simulink model "f16_6dof3"  (R2020b)
settings: Solver=VariableStepAuto  StartTime=0.0  StopTime=100  RelTol=1e-3
values from neighbouring files (symbols this model uses):
  b = 9.144    [f16_script3.m]
  chord = 3.45    [f16_script3.m]
  d_r = 0    [f16_script3.m]
  d_SB = 0    [f16_script3.m]
  h_ref = 0    [f16_script3.m]
  Mass = 9300    [f16_script3.m]
  phi_c = 10    [f16_script3.m]
  S = 27.88    [f16_script3.m]
  V_c = 153    [f16_script3.m]
  X_cg = 0.35    [f16_script3.m]
  X_cg_ref = 0.35    [f16_script3.m]
undefined symbols (not defined in the file or in its folder): block, Earth, f16, f16_database, WGS84
libraries: simulink_extras x7, slpidlib x4, aerolibfltsims x2, shared6dof x1, aerolibatmos2 x1, aerolibasang x1, aerolibtransform2 x1
(part 1 of 2)
settings Model: Creator=celal  LastModifiedBy=celal

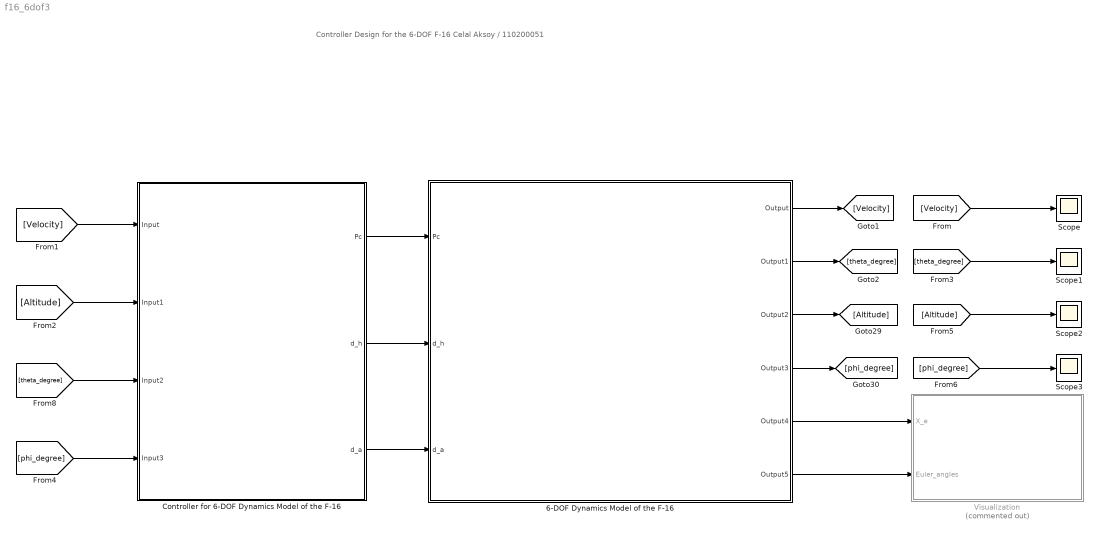
== system f16_6dof3 ==
  note: Controller Design for the 6-DOF F-16
      |
      | Celal Aksoy / 110200051
  " 6-DOF Dynamics Model of the F-16" : Subsystem
  Controller for 6-DOF Dynamics Model of the F-16 : Subsystem
  Scope{,1..3} (4 alike) : Scope
  Visualization : Subsystem  Commented=on
  wires:
  " 6-DOF Dynamics Model of the F-16"/1(Output) -> [Velocity]
  " 6-DOF Dynamics Model of the F-16"/2(Output1) -> [theta_degree]
  " 6-DOF Dynamics Model of the F-16"/3(Output2) -> [Altitude]
  " 6-DOF Dynamics Model of the F-16"/4(Output3) -> [phi_degree]
  [Velocity] -> Controller for 6-DOF Dynamics Model of the F-16/1(Input)
  [theta_degree] -> Controller for 6-DOF Dynamics Model of the F-16/3(Input2)
  [phi_degree] -> Controller for 6-DOF Dynamics Model of the F-16/4(Input3)
  [Altitude] -> Controller for 6-DOF Dynamics Model of the F-16/2(Input1)
  [Velocity] -> Scope/1
  [Altitude] -> Scope2/1
  [phi_degree] -> Scope3/1
  [theta_degree] -> Scope1/1
  Controller for 6-DOF Dynamics Model of the F-16/2(d_h) -> " 6-DOF Dynamics Model of the F-16"/2(d_h)
  Controller for 6-DOF Dynamics Model of the F-16/1(Pc) -> " 6-DOF Dynamics Model of the F-16"/1(Pc)
  Controller for 6-DOF Dynamics Model of the F-16/3(d_a) -> " 6-DOF Dynamics Model of the F-16"/3(d_a)
  " 6-DOF Dynamics Model of the F-16"/5(Output4) -> Visualization/1(X_e)
  " 6-DOF Dynamics Model of the F-16"/6(Output5) -> Visualization/2(Euler_angles)

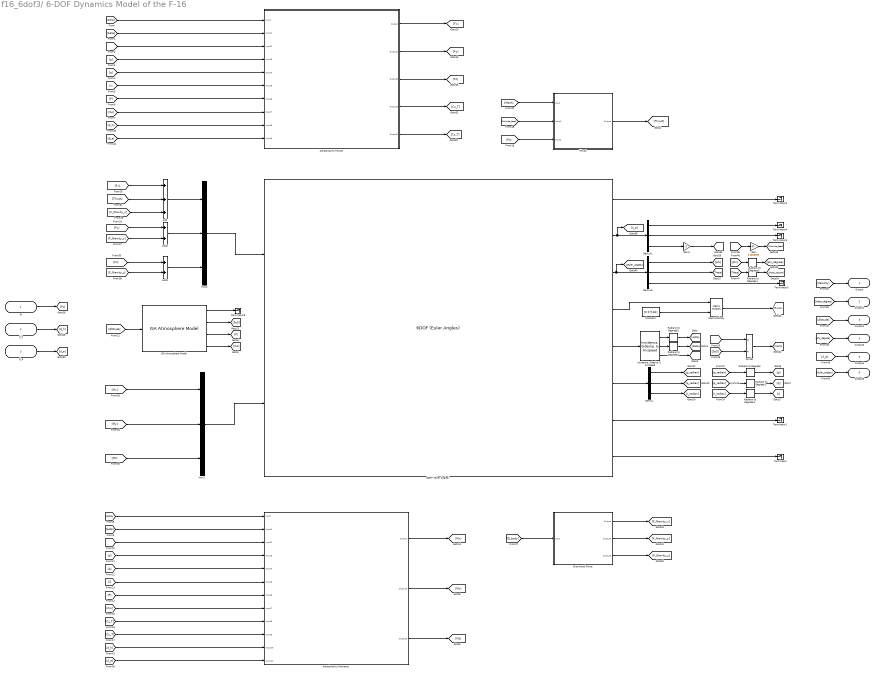
== system f16_6dof3/ 6-DOF Dynamics Model of the F-16 ==
  Pc : Inport
  d_h : Inport  Port=2
  d_a : Inport  Port=3
  6DOF (Euler Angles) : shared6dof/6DOF (Euler Angles)  units=Metric (MKS)  mtype=Fixed  rep=Euler Angles  xme_0=[0, 0, -3048 ]  Vm_0=[131.2, 0, 0]  eul_0=[0, 0, 0]  pm_0=[0, 0, 0]  mass_0=9300  mass_e=0.5  mass_f=2.0  inertia=I  inertia_e=eye(3)  inertia_f=2*eye(3)  k_quat=1.0  vre_flag=on  abi_flag=off  aMode=0  xme_statename=''  Vm_statename=''  eul_statename=''  quat_statename=''  pm_statename=''  mass_statename=''
      settings: SourceProductBaseCode=AE,PW,MT,UV,VE,VP
  Add : Sum  Inputs=+++
  Add1 : Sum
  Add3 : Sum
  Aerodynamic Forces : Subsystem
  Aerodynamic Moments : Subsystem
  Constant : Constant  Value=[0 0 9.81]
  Demux : Demux  Outputs=3
  Demux1 : Demux  Outputs=3
  Demux3 : Demux  Outputs=3
  Divide : Product  Inputs=*/
  Gain : Gain  Gain=3.2808399
  Gain1 : Gain  Gain=-1
  Gravitional Force : Subsystem
  ISA Atmosphere Model : aerolibatmos2/ISA Atmosphere Model  custom=off  g=9.80665  gamma=1.4  R=287.0531  L=0.0065  h_trop=11000  h_strat=20000  rho0=1.225  P0=101325  T0=288.15  h0=0
  "Incidence, Sideslip, & Airspeed" : aerolibasang/Incidence, Sideslip, & Airspeed
  MatrixMultiply : Product  Multiplication=Matrix(*)
  Mux1 : Mux  Inputs=3
  Mux2 : Mux  Inputs=3
  Radians to Degrees{,1..6} (7 alike) : simulink_extras/Transformations/Radians to Degrees
  Terminator{,1..5,8} (7 alike) : Terminator
  Thrust : Subsystem
  Output : Outport
  Output1 : Outport  Port=2
  Output2 : Outport  Port=3
  Output3 : Outport  Port=4
  Output4 : Outport  Port=5
  Output5 : Outport  Port=6
  wires:
  Gain/1 -> [Altitude_feet]
  [P] -> Aerodynamic Forces/7(Input6)
  6DOF (Euler Angles)/5 -> "Incidence, Sideslip, & Airspeed"/1
  [beta] -> Aerodynamic Forces/2(Input1)
  [beta] -> Aerodynamic Moments/2(Input1)
  Aerodynamic Moments/1(Output) -> [Mx]
  ISA Atmosphere Model/4 -> [rho]
  [Mz] -> Mux1/3
  [alpha] -> Aerodynamic Forces/1(Input)
  Demux/1 -> [p_radian]
  [r] -> Aerodynamic Forces/6(Input5)
  Demux3/2 -> [Theta]
  Mux1/1 -> 6DOF (Euler Angles)/2
  Demux/3 -> [r_radian]
  Demux/2 -> [q_radian]
  [r] -> Aerodynamic Moments/6(Input5)
  Constant/1 -> MatrixMultiply/2
  6DOF (Euler Angles)/7 -> Terminator1/1
  [rho] -> Aerodynamic Forces/8(Input7)
  [Altitude_feet] -> Thrust/2(Input1)
  ISA Atmosphere Model/3 -> [P]
  6DOF (Euler Angles)/6 -> Demux/1
  [r_radian] -> Radians to Degrees2/1
  [p] -> Aerodynamic Forces/4(Input3)
  ISA Atmosphere Model/2 -> [SoS]
  [G_body] -> Gravitional Force/1(Input)
  [Mach] -> Thrust/1(Input)
  Demux1/1 -> Terminator4/1
  [rho] -> Aerodynamic Moments/8(Input7)
  Aerodynamic Forces/1(Output) -> [Fx]
  [P] -> Aerodynamic Moments/7(Input6)
  [Cz_T] -> Aerodynamic Moments/9(Input8)
  Aerodynamic Moments/3(Output2) -> [Mz]
  [p_radian] -> Radians to Degrees/1
  Thrust/1(Output) -> [Thrust]
  [alpha] -> Aerodynamic Moments/1(Input)
  Aerodynamic Moments/2(Output1) -> [My]
  [Velocity] -> Aerodynamic Moments/3(Input2)
  Aerodynamic Forces/3(Output2) -> [Fz]
  [q] -> Aerodynamic Forces/5(Input4)
  Radians to Degrees2/1 -> [r]
  [q_radian] -> Radians to Degrees1/1
  Radians to Degrees1/1 -> [q]
  [p] -> Aerodynamic Moments/4(Input3)
  6DOF (Euler Angles)/2 -> [X_e], Demux1/1
  MatrixMultiply/1 -> [G_body]
  Divide/1 -> [Mach]
  6DOF (Euler Angles)/3 -> [Euler_angles], Demux3/1
  6DOF (Euler Angles)/1 -> Terminator2/1
  6DOF (Euler Angles)/8 -> Terminator/1
  Demux1/2 -> Terminator5/1
  [Altitude] -> ISA Atmosphere Model/1
  [SoS] -> Divide/2
  [Cy_T] -> Aerodynamic Moments/10(Input9)
  [q] -> Aerodynamic Moments/5(Input4)
  Aerodynamic Forces/2(Output1) -> [Fy]
  [Mx] -> Mux1/1
  ISA Atmosphere Model/1 -> Terminator8/1
  [Velocity] -> Aerodynamic Forces/3(Input2)
  [My] -> Mux1/2
  [Altitude] -> Gain/1
  Radians to Degrees/1 -> [p]
  6DOF (Euler Angles)/4 -> MatrixMultiply/1
  [Velocity] -> Divide/1
  Demux3/3 -> Terminator3/1
  Demux3/1 -> [phi]
  [Pc] -> Thrust/3(Input2)
  Gravitional Force/2(Output1) -> [F_Gravity_y]
  Gravitional Force/3(Output2) -> [F_Gravity_z]
  Gravitional Force/1(Output) -> [F_Gravity_x]
  Pc/1 -> [Pc]
  [Velocity] -> Output/1
  d_h/1 -> [d_h]
  [d_h] -> Aerodynamic Forces/9(Input8)
  [d_h] -> Aerodynamic Moments/11(Input10)
  [Altitude] -> Output2/1
  [phi_degree] -> Output3/1
  d_a/1 -> [d_a]
  [d_a] -> Aerodynamic Forces/10(Input9)
  [d_a] -> Aerodynamic Moments/12(Input11)
  Aerodynamic Forces/4(Output3) -> [Cz_T]
  Aerodynamic Forces/5(Output4) -> [Cy_T]
  [phi] -> Radians to Degrees3/1
  [Theta] -> Radians to Degrees4/1
  Radians to Degrees3/1 -> [phi_degree]
  Radians to Degrees4/1 -> [theta_degree]
  [theta_degree] -> Output1/1
  Gain1/1 -> [Altitude]
  Mux2/1 -> 6DOF (Euler Angles)/1
  [Fx] -> Add/1
  [Thrust] -> Add/2
  [F_Gravity_x] -> Add/3
  Add/1 -> Mux2/1
  [Fy] -> Add1/1
  [F_Gravity_y] -> Add1/2
  Add1/1 -> Mux2/2
  Add3/1 -> Mux2/3
  [Fz] -> Add3/1
  [F_Gravity_z] -> Add3/2
  Demux1/3 -> Gain1/1
  "Incidence, Sideslip, & Airspeed"/1 -> Radians to Degrees5/1
  "Incidence, Sideslip, & Airspeed"/2 -> Radians to Degrees6/1
  Radians to Degrees5/1 -> [alpha]
  Radians to Degrees6/1 -> [beta]
  "Incidence, Sideslip, & Airspeed"/3 -> [Velocity]
  [X_e] -> Output4/1
  [Euler_angles] -> Output5/1

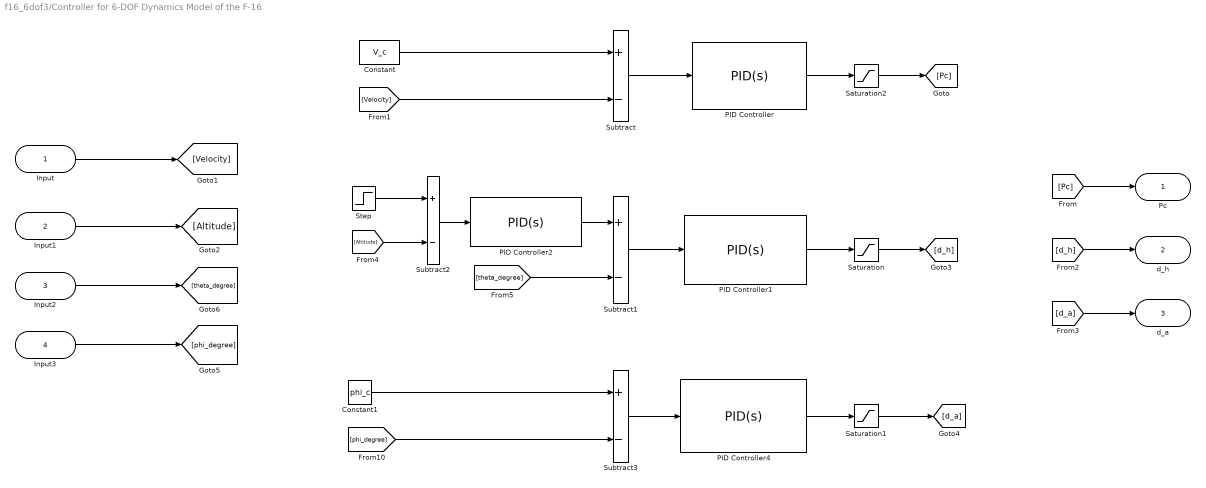
== system f16_6dof3/Controller for 6-DOF Dynamics Model of the F-16 ==
  Input : Inport
  Input1 : Inport  Port=2
  Input2 : Inport  Port=3
  Input3 : Inport  Port=4
  Constant : Constant  Value=V_c
  Constant1 : Constant  Value=phi_c
  PID Controller : slpidlib/PID Controller  Controller=PID  Form=Parallel  TimeDomain=Continuous-time  UseExternalTs=off  SampleTime=-1  IntegratorMethod=Forward Euler  FilterMethod=Forward Euler  ControllerParametersSource=internal  P=70  I=15  D=50  UseFilter=on  N=10  TunerSelectOption=Transfer Function Based (PID Tuner App)  InitialConditionSource=internal  InitialConditionForIntegrator=0  InitialConditionForFilter=0  DifferentiatorICPrevScaledInput=0  ExternalReset=none  TrackingMode=off  Kt=1  LimitOutput=off  SatLimitsSource=internal  UpperSaturationLimit=inf  LowerSaturationLimit=-inf  LinearizeAsGain=on  AntiWindupMode=none  Kb=1  POutMin=[]  POutMax=[]  IOutMin=[]  IOutMax=[]  DOutMin=[]  DOutMax=[]  NOutMin=[]  NOutMax=[]  SumOutMin=[]  SumOutMax=[]  SaturationOutMin=[]  SaturationOutMax=[]  PParamMin=[]  PParamMax=[]  IParamMin=[]  IParamMax=[]  DParamMin=[]  DParamMax=[]  NParamMin=[]  NParamMax=[]  KbParamMin=[]  KbParamMax=[]  KtParamMin=[]  KtParamMax=[]  KbOutMin=[]  KbOutMax=[]  KtOutMin=[]  KtOutMax=[]  IntegratorOutMin=[]  IntegratorOutMax=[]  FilterOutMin=[]  FilterOutMax=[]  SumI1OutMin=[]  SumI1OutMax=[]  SumI2OutMin=[]  SumI2OutMax=[]  SumI3OutMin=[]  SumI3OutMax=[]  SumI4OutMin=[]  SumI4OutMax=[]  SumDOutMin=[]  SumDOutMax=[]  DifferentiatorOutMin=[]  DifferentiatorOutMax=[]  FilterDiffOutCoefMin=[]  FilterDiffOutCoefMax=[]  ReciprocalOutMin=[]  ReciprocalOutMax=[]  SumDenOutMin=[]  SumDenOutMax=[]  SumNumOutMin=[]  SumNumOutMax=[]  DivideOutMin=[]  DivideOutMax=[]  UdiffTsProdOutMin=[]  UdiffTsProdOutMax=[]  NTsProdOutMin=[]  NTsProdOutMax=[]  UintegralTsProdOutMin=[]  UintegralTsProdOutMax=[]  UngainTsProdOutMin=[]  UngainTsProdOutMax=[]  IntegratorContinuousStateAttributes=''  IntegratorStateMustResolveToSignalObject=off  IntegratorRTWStateStorageClass=Auto  FilterContinuousStateAttributes=''  FilterStateMustResolveToSignalObject=off  FilterRTWStateStorageClass=Auto  ParallelPVariant=InternalParameters  IdealPVariant=Disabled  IVariant=InternalParameters  DVariant=InternalParameters  IntegratorVariant=Continuous  SatVariant=Disabled  AWVariant=Passthrough  PCopyVariant=Disabled  TRVariant=Disabled  FdbkBlocksVariant=Forward  IdealPFdbkVariant=Disabled  SatFdbkVariant=Disabled  DerivativeFilterVariant=ContFilter  NVariant=InternalParameters  NCopyVariant=Disabled  FilterICVariant=InternalICsFilter  IntegratorICVariant=InternalICs  ExternalResetVariant=Disabled  TRSumVariant=Passthrough  SumFdbkVariant=Disabled  SumVariant=Sum_PID  TsampFilterVariant=InternalTs  TsampNgainVariant=Passthrough  TsampIntegralVariant=Passthrough  ExternalSaturationOutDataTypeStr=Inherit: Same as second input  mask(PID 1dof){}
      mask Display:
      | % This is a new mask on top of the base mask.
      | % Use "View base mask" link below to see the base mask.
      | disp("Velocity Hold Controller");
  PID Controller1 : slpidlib/PID Controller  Controller=PID  Form=Parallel  TimeDomain=Continuous-time  UseExternalTs=off  SampleTime=-1  IntegratorMethod=Forward Euler  FilterMethod=Forward Euler  ControllerParametersSource=internal  P=-6e-07  I=-3e-10  D=-12e-7  UseFilter=on  N=2.9  TunerSelectOption=Transfer Function Based (PID Tuner App)  InitialConditionSource=internal  InitialConditionForIntegrator=0  InitialConditionForFilter=0  DifferentiatorICPrevScaledInput=0  ExternalReset=none  TrackingMode=off  Kt=1  LimitOutput=off  SatLimitsSource=internal  UpperSaturationLimit=inf  LowerSaturationLimit=-inf  LinearizeAsGain=on  AntiWindupMode=none  Kb=1  POutMin=[]  POutMax=[]  IOutMin=[]  IOutMax=[]  DOutMin=[]  DOutMax=[]  NOutMin=[]  NOutMax=[]  SumOutMin=[]  SumOutMax=[]  SaturationOutMin=[]  SaturationOutMax=[]  PParamMin=[]  PParamMax=[]  IParamMin=[]  IParamMax=[]  DParamMin=[]  DParamMax=[]  NParamMin=[]  NParamMax=[]  KbParamMin=[]  KbParamMax=[]  KtParamMin=[]  KtParamMax=[]  KbOutMin=[]  KbOutMax=[]  KtOutMin=[]  KtOutMax=[]  IntegratorOutMin=[]  IntegratorOutMax=[]  FilterOutMin=[]  FilterOutMax=[]  SumI1OutMin=[]  SumI1OutMax=[]  SumI2OutMin=[]  SumI2OutMax=[]  SumI3OutMin=[]  SumI3OutMax=[]  SumI4OutMin=[]  SumI4OutMax=[]  SumDOutMin=[]  SumDOutMax=[]  DifferentiatorOutMin=[]  DifferentiatorOutMax=[]  FilterDiffOutCoefMin=[]  FilterDiffOutCoefMax=[]  ReciprocalOutMin=[]  ReciprocalOutMax=[]  SumDenOutMin=[]  SumDenOutMax=[]  SumNumOutMin=[]  SumNumOutMax=[]  DivideOutMin=[]  DivideOutMax=[]  UdiffTsProdOutMin=[]  UdiffTsProdOutMax=[]  NTsProdOutMin=[]  NTsProdOutMax=[]  UintegralTsProdOutMin=[]  UintegralTsProdOutMax=[]  UngainTsProdOutMin=[]  UngainTsProdOutMax=[]  IntegratorContinuousStateAttributes=''  IntegratorStateMustResolveToSignalObject=off  IntegratorRTWStateStorageClass=Auto  FilterContinuousStateAttributes=''  FilterStateMustResolveToSignalObject=off  FilterRTWStateStorageClass=Auto  ParallelPVariant=InternalParameters  IdealPVariant=Disabled  IVariant=InternalParameters  DVariant=InternalParameters  IntegratorVariant=Continuous  SatVariant=Disabled  AWVariant=Passthrough  PCopyVariant=Disabled  TRVariant=Disabled  FdbkBlocksVariant=Forward  IdealPFdbkVariant=Disabled  SatFdbkVariant=Disabled  DerivativeFilterVariant=ContFilter  NVariant=InternalParameters  NCopyVariant=Disabled  FilterICVariant=InternalICsFilter  IntegratorICVariant=InternalICs  ExternalResetVariant=Disabled  TRSumVariant=Passthrough  SumFdbkVariant=Disabled  SumVariant=Sum_PID  TsampFilterVariant=InternalTs  TsampNgainVariant=Passthrough  TsampIntegralVariant=Passthrough  ExternalSaturationOutDataTypeStr=Inherit: Same as second input  mask(PID 1dof){}
      mask Display:
      | % This is a new mask on top of the base mask.
      | % Use "View base mask" link below to see the base mask.
      | disp("Pitch-Attitude Hold Controller")
  PID Controller2 : slpidlib/PID Controller  Controller=PID  Form=Parallel  TimeDomain=Continuous-time  UseExternalTs=off  SampleTime=-1  IntegratorMethod=Forward Euler  FilterMethod=Forward Euler  ControllerParametersSource=internal  P=10000000  I=50000  D=1000  UseFilter=on  N=1e-03  TunerSelectOption=Transfer Function Based (PID Tuner App)  InitialConditionSource=internal  InitialConditionForIntegrator=0  InitialConditionForFilter=0  DifferentiatorICPrevScaledInput=0  ExternalReset=none  TrackingMode=off  Kt=1  LimitOutput=off  SatLimitsSource=internal  UpperSaturationLimit=inf  LowerSaturationLimit=-inf  LinearizeAsGain=on  AntiWindupMode=none  Kb=1  POutMin=[]  POutMax=[]  IOutMin=[]  IOutMax=[]  DOutMin=[]  DOutMax=[]  NOutMin=[]  NOutMax=[]  SumOutMin=[]  SumOutMax=[]  SaturationOutMin=[]  SaturationOutMax=[]  PParamMin=[]  PParamMax=[]  IParamMin=[]  IParamMax=[]  DParamMin=[]  DParamMax=[]  NParamMin=[]  NParamMax=[]  KbParamMin=[]  KbParamMax=[]  KtParamMin=[]  KtParamMax=[]  KbOutMin=[]  KbOutMax=[]  KtOutMin=[]  KtOutMax=[]  IntegratorOutMin=[]  IntegratorOutMax=[]  FilterOutMin=[]  FilterOutMax=[]  SumI1OutMin=[]  SumI1OutMax=[]  SumI2OutMin=[]  SumI2OutMax=[]  SumI3OutMin=[]  SumI3OutMax=[]  SumI4OutMin=[]  SumI4OutMax=[]  SumDOutMin=[]  SumDOutMax=[]  DifferentiatorOutMin=[]  DifferentiatorOutMax=[]  FilterDiffOutCoefMin=[]  FilterDiffOutCoefMax=[]  ReciprocalOutMin=[]  ReciprocalOutMax=[]  SumDenOutMin=[]  SumDenOutMax=[]  SumNumOutMin=[]  SumNumOutMax=[]  DivideOutMin=[]  DivideOutMax=[]  UdiffTsProdOutMin=[]  UdiffTsProdOutMax=[]  NTsProdOutMin=[]  NTsProdOutMax=[]  UintegralTsProdOutMin=[]  UintegralTsProdOutMax=[]  UngainTsProdOutMin=[]  UngainTsProdOutMax=[]  IntegratorContinuousStateAttributes=''  IntegratorStateMustResolveToSignalObject=off  IntegratorRTWStateStorageClass=Auto  FilterContinuousStateAttributes=''  FilterStateMustResolveToSignalObject=off  FilterRTWStateStorageClass=Auto  ParallelPVariant=InternalParameters  IdealPVariant=Disabled  IVariant=InternalParameters  DVariant=InternalParameters  IntegratorVariant=Continuous  SatVariant=Disabled  AWVariant=Passthrough  PCopyVariant=Disabled  TRVariant=Disabled  FdbkBlocksVariant=Forward  IdealPFdbkVariant=Disabled  SatFdbkVariant=Disabled  DerivativeFilterVariant=ContFilter  NVariant=InternalParameters  NCopyVariant=Disabled  FilterICVariant=InternalICsFilter  IntegratorICVariant=InternalICs  ExternalResetVariant=Disabled  TRSumVariant=Passthrough  SumFdbkVariant=Disabled  SumVariant=Sum_PID  TsampFilterVariant=InternalTs  TsampNgainVariant=Passthrough  TsampIntegralVariant=Passthrough  ExternalSaturationOutDataTypeStr=Inherit: Same as second input  mask(PID 1dof){}
      mask Display:
      | % This is a new mask on top of the base mask.
      | % Use "View base mask" link below to see the base mask.
      | disp("Altitude Hold Controller");
  PID Controller4 : slpidlib/PID Controller  Controller=PID  Form=Parallel  TimeDomain=Continuous-time  UseExternalTs=off  SampleTime=-1  IntegratorMethod=Forward Euler  FilterMethod=Forward Euler  ControllerParametersSource=internal  P=-15  I=-0.010  D=-0.001  UseFilter=on  N=0.6  TunerSelectOption=Transfer Function Based (PID Tuner App)  InitialConditionSource=internal  InitialConditionForIntegrator=0  InitialConditionForFilter=0  DifferentiatorICPrevScaledInput=0  ExternalReset=none  TrackingMode=off  Kt=1  LimitOutput=off  SatLimitsSource=internal  UpperSaturationLimit=inf  LowerSaturationLimit=-inf  LinearizeAsGain=on  AntiWindupMode=none  Kb=1  POutMin=[]  POutMax=[]  IOutMin=[]  IOutMax=[]  DOutMin=[]  DOutMax=[]  NOutMin=[]  NOutMax=[]  SumOutMin=[]  SumOutMax=[]  SaturationOutMin=[]  SaturationOutMax=[]  PParamMin=[]  PParamMax=[]  IParamMin=[]  IParamMax=[]  DParamMin=[]  DParamMax=[]  NParamMin=[]  NParamMax=[]  KbParamMin=[]  KbParamMax=[]  KtParamMin=[]  KtParamMax=[]  KbOutMin=[]  KbOutMax=[]  KtOutMin=[]  KtOutMax=[]  IntegratorOutMin=[]  IntegratorOutMax=[]  FilterOutMin=[]  FilterOutMax=[]  SumI1OutMin=[]  SumI1OutMax=[]  SumI2OutMin=[]  SumI2OutMax=[]  SumI3OutMin=[]  SumI3OutMax=[]  SumI4OutMin=[]  SumI4OutMax=[]  SumDOutMin=[]  SumDOutMax=[]  DifferentiatorOutMin=[]  DifferentiatorOutMax=[]  FilterDiffOutCoefMin=[]  FilterDiffOutCoefMax=[]  ReciprocalOutMin=[]  ReciprocalOutMax=[]  SumDenOutMin=[]  SumDenOutMax=[]  SumNumOutMin=[]  SumNumOutMax=[]  DivideOutMin=[]  DivideOutMax=[]  UdiffTsProdOutMin=[]  UdiffTsProdOutMax=[]  NTsProdOutMin=[]  NTsProdOutMax=[]  UintegralTsProdOutMin=[]  UintegralTsProdOutMax=[]  UngainTsProdOutMin=[]  UngainTsProdOutMax=[]  IntegratorContinuousStateAttributes=''  IntegratorStateMustResolveToSignalObject=off  IntegratorRTWStateStorageClass=Auto  FilterContinuousStateAttributes=''  FilterStateMustResolveToSignalObject=off  FilterRTWStateStorageClass=Auto  ParallelPVariant=InternalParameters  IdealPVariant=Disabled  IVariant=InternalParameters  DVariant=InternalParameters  IntegratorVariant=Continuous  SatVariant=Disabled  AWVariant=Passthrough  PCopyVariant=Disabled  TRVariant=Disabled  FdbkBlocksVariant=Forward  IdealPFdbkVariant=Disabled  SatFdbkVariant=Disabled  DerivativeFilterVariant=ContFilter  NVariant=InternalParameters  NCopyVariant=Disabled  FilterICVariant=InternalICsFilter  IntegratorICVariant=InternalICs  ExternalResetVariant=Disabled  TRSumVariant=Passthrough  SumFdbkVariant=Disabled  SumVariant=Sum_PID  TsampFilterVariant=InternalTs  TsampNgainVariant=Passthrough  TsampIntegralVariant=Passthrough  ExternalSaturationOutDataTypeStr=Inherit: Same as second input  mask(PID 1dof){}
      mask Display:
      | % This is a new mask on top of the base mask.
      | % Use "View base mask" link below to see the base mask.
      | disp("Roll-Angle Hold Controller")
  Saturation : Saturate  UpperLimit=25  LowerLimit=-25
  Saturation1 : Saturate  UpperLimit=20  LowerLimit=-20
  Saturation2 : Saturate  UpperLimit=100  LowerLimit=0
  Step : Step  Time=60  Before=10100*0.3048  After=9090*0.3048  SampleTime=0
  Subtract{,1..3} (4 alike) : Sum  Inputs=+-
  Pc : Outport
  d_h : Outport  Port=2
  d_a : Outport  Port=3
  wires:
  Constant/1 -> Subtract/1
  Saturation/1 -> [d_h]
  PID Controller4/1 -> Saturation1/1
  Subtract3/1 -> PID Controller4/1
  Saturation1/1 -> [d_a]
  PID Controller2/1 -> Subtract1/1
  Subtract2/1 -> PID Controller2/1
  PID Controller1/1 -> Saturation/1
  [phi_degree] -> Subtract3/2
  Step/1 -> Subtract2/1
  Subtract/1 -> PID Controller/1
  [Altitude] -> Subtract2/2
  Constant1/1 -> Subtract3/1
  Subtract1/1 -> PID Controller1/1
  [theta_degree] -> Subtract1/2
  [Velocity] -> Subtract/2
  Saturation2/1 -> [Pc]
  PID Controller/1 -> Saturation2/1
  Input3/1 -> [phi_degree]
  Input2/1 -> [theta_degree]
  Input1/1 -> [Altitude]
  Input/1 -> [Velocity]
  [Pc] -> Pc/1
  [d_h] -> d_h/1
  [d_a] -> d_a/1

== system f16_6dof3/Visualization ==
  X_e : Inport
  Euler_angles : Inport  Port=2
  Constant : Constant  Value=h_ref
  Demux : Demux  Outputs=3
  Demux1 : Demux  Outputs=2
  Flat Earth to LLA : aerolibtransform2/Flat Earth to LLA  units=Metric (MKS)  ptype=Earth (WGS84)  F=1/298.257223563  R=6378137  refPosPort=off  LL0=[0 10]  psi=0
  FlightGear Preconfigured 6DoF Animation : aerolibfltsims/FlightGear Preconfigured 6DoF Animation  xFlightGearVersion=v2019.1  DestinationIpAddress=127.0.0.1  DestinationPort=5502  SampleTime=1/30  packetVersion=24
  Generate Run Script : aerolibfltsims/Generate Run Script  Architecture=Default  dataFlow=Send  GeometryModelName=f16-block-30  AirportId=KSFO  RunwayId=10L  InitialAltitude=7224  InitialHeading=113  OffsetDistance=4.72  OffsetAzimuth=0  InstallScenery=off  DisableShaders=off  OriginAddress=127.0.0.1  DestinationPort=5502  OriginPort=5505  LocalAddress=127.0.0.1  OutputFileName=runfg.bat  FlightGearBaseDirectory=C:\Program Files\FlightGear 2020.3
  Mux : Mux  Inputs=6
  wires:
  Constant/1 -> Flat Earth to LLA/2
  Mux/1 -> FlightGear Preconfigured 6DoF Animation/1
  Demux/1 -> Mux/4
  [X_e] -> Flat Earth to LLA/1
  Demux/2 -> Mux/5
  [Euler_angles] -> Demux/1
  Demux/3 -> Mux/6
  X_e/1 -> [X_e]
  Euler_angles/1 -> [Euler_angles]
  Flat Earth to LLA/1 -> Demux1/1
  Demux1/2 -> Mux/1
  Demux1/1 -> Mux/2
  Flat Earth to LLA/2 -> Mux/3

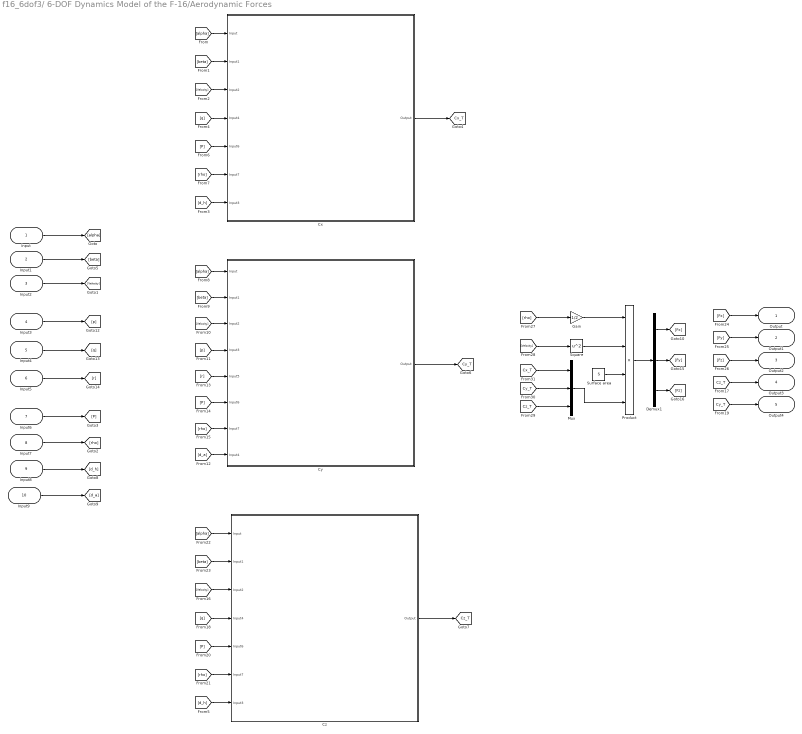
== system f16_6dof3/ 6-DOF Dynamics Model of the F-16/Aerodynamic Forces ==
  Input : Inport
  Input1 : Inport  Port=2
  Input2 : Inport  Port=3
  Input3 : Inport  Port=4
  Input4 : Inport  Port=5
  Input5 : Inport  Port=6
  Input6 : Inport  Port=7
  Input7 : Inport  Port=8
  Input8 : Inport  Port=9
  Input9 : Inport  Port=10
  Cx : Subsystem
  Cy : Subsystem
  Cz : Subsystem
  Demux1 : Demux  Outputs=3
  Gain : Gain  Gain=1/2
  Mux : Mux  Inputs=3
  Product : Product  Inputs=4
  Square : Math  Operator=square  SaturateOnIntegerOverflow=on
  Surface area : Constant  Value=S
  Output : Outport
  Output1 : Outport  Port=2
  Output2 : Outport  Port=3
  Output3 : Outport  Port=4
  Output4 : Outport  Port=5
  tag scope: Cx_T=global, Cy_T=global, Cz_T=global
  wires:
  Input/1 -> [alpha]
  Input1/1 -> [beta]
  Input2/1 -> [Velocity]
  Input6/1 -> [P]
  Input7/1 -> [rho]
  Input5/1 -> [r]
  Input4/1 -> [q]
  Input3/1 -> [p]
  [alpha] -> Cx/1(Input)
  [beta] -> Cx/2(Input1)
  [Velocity] -> Cx/3(Input2)
  [q] -> Cx/4(Input4)
  [P] -> Cx/5(Input6)
  [rho] -> Cx/6(Input7)
  Cx/1(Output) -> [Cx_T]
  Cy/1(Output) -> [Cy_T]
  [P] -> Cy/6(Input6)
  [Velocity] -> Cy/3(Input2)
  [rho] -> Cy/7(Input7)
  [alpha] -> Cy/1(Input)
  [beta] -> Cy/2(Input1)
  [p] -> Cy/4(Input3)
  [r] -> Cy/5(Input5)
  [q] -> Cz/4(Input4)
  [beta] -> Cz/2(Input1)
  [alpha] -> Cz/1(Input)
  [rho] -> Cz/6(Input7)
  [Velocity] -> Cz/3(Input2)
  [P] -> Cz/5(Input6)
  Cz/1(Output) -> [Cz_T]
  [Fx] -> Output/1
  [Fy] -> Output1/1
  [Fz] -> Output2/1
  Demux1/3 -> [Fz]
  Surface area/1 -> Product/3
  Demux1/1 -> [Fx]
  Square/1 -> Product/2
  Gain/1 -> Product/1
  [Velocity] -> Square/1
  [Cx_T] -> Mux/1
  [rho] -> Gain/1
  Demux1/2 -> [Fy]
  Product/1 -> Demux1/1
  Mux/1 -> Product/4
  [Cy_T] -> Mux/2
  [Cz_T] -> Mux/3
  Input8/1 -> [d_h]
  [d_h] -> Cx/7(Input3)
  [d_h] -> Cz/7(Input3)
  Input9/1 -> [d_a]
  [d_a] -> Cy/8(Input4)
  [Cz_T] -> Output3/1
  [Cy_T] -> Output4/1

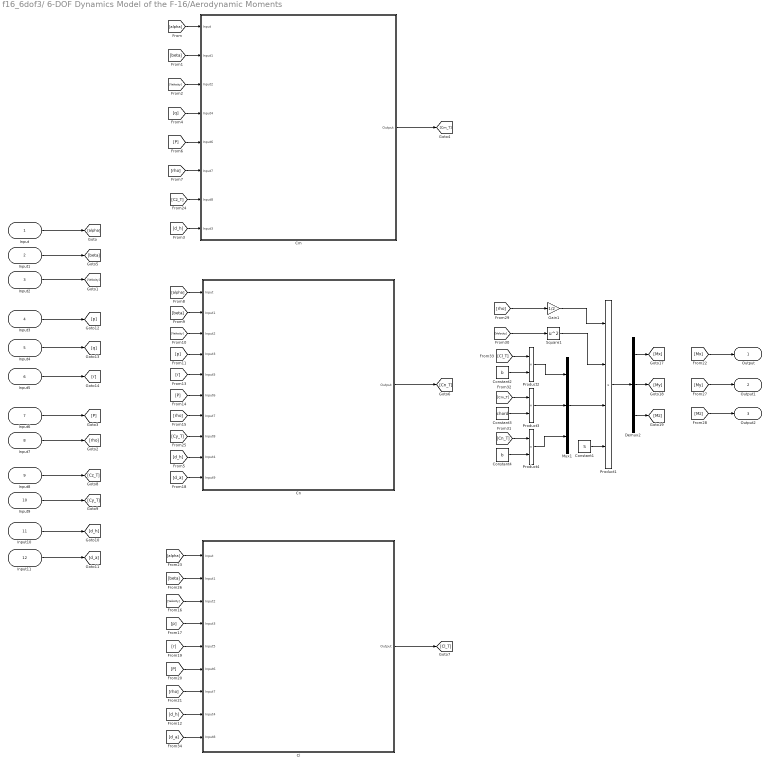
== system f16_6dof3/ 6-DOF Dynamics Model of the F-16/Aerodynamic Moments ==
  Input : Inport
  Input1 : Inport  Port=2
  Input2 : Inport  Port=3
  Input3 : Inport  Port=4
  Input4 : Inport  Port=5
  Input5 : Inport  Port=6
  Input6 : Inport  Port=7
  Input7 : Inport  Port=8
  Input8 : Inport  Port=9
  Input9 : Inport  Port=10
  Input10 : Inport  Port=11
  Input11 : Inport  Port=12
  "Cl " : Subsystem
  Cm : Subsystem
  Cn : Subsystem
  Constant1 : Constant  Value=S
  Constant2 : Constant  Value=b
  Constant3 : Constant  Value=chord
  Constant4 : Constant  Value=b
  Demux2 : Demux  Outputs=3
  Gain1 : Gain  Gain=1/2
  Mux1 : Mux  Inputs=3
  Product1 : Product  Inputs=4
  Product2 : Product
  Product3 : Product
  Product4 : Product
  Square1 : Math  Operator=square  SaturateOnIntegerOverflow=on
  Output : Outport
  Output1 : Outport  Port=2
  Output2 : Outport  Port=3
  wires:
  [r] -> Cn/5(Input5)
  [p] -> Cn/4(Input3)
  [beta] -> Cn/2(Input1)
  [alpha] -> Cn/1(Input)
  [rho] -> Cn/7(Input7)
  [Velocity] -> Cn/3(Input2)
  [P] -> Cn/6(Input6)
  Cn/1(Output) -> [Cn_T]
  [rho] -> Cm/6(Input7)
  [P] -> Cm/5(Input6)
  [q] -> Cm/4(Input4)
  [Velocity] -> Cm/3(Input2)
  [beta] -> Cm/2(Input1)
  [alpha] -> Cm/1(Input)
  Input3/1 -> [p]
  Input4/1 -> [q]
  Input5/1 -> [r]
  Input7/1 -> [rho]
  Input6/1 -> [P]
  Input2/1 -> [Velocity]
  Input1/1 -> [beta]
  Input/1 -> [alpha]
  Input8/1 -> [Cz_T]
  [Cz_T] -> Cm/7(Input8)
  Cm/1(Output) -> [Cm_T]
  Input9/1 -> [Cy_T]
  [Cy_T] -> Cn/8(Input8)
  "Cl "/1(Output) -> [Cl_T]
  [P] -> "Cl "/6(Input6)
  [Velocity] -> "Cl "/3(Input2)
  [rho] -> "Cl "/7(Input7)
  [alpha] -> "Cl "/1(Input)
  [beta] -> "Cl "/2(Input1)
  [p] -> "Cl "/4(Input3)
  [r] -> "Cl "/5(Input5)
  [Mx] -> Output/1
  [My] -> Output1/1
  [Mz] -> Output2/1
  Demux2/3 -> [Mz]
  Product3/1 -> Mux1/2
  Gain1/1 -> Product1/1
  [rho] -> Gain1/1
  Product4/1 -> Mux1/3
  Square1/1 -> Product1/2
  [Velocity] -> Square1/1
  Product1/1 -> Demux2/1
  [Cl_T] -> Product2/1
  Constant3/1 -> Product3/2
  Product2/1 -> Mux1/1
  Constant1/1 -> Product1/4
  Demux2/1 -> [Mx]
  Demux2/2 -> [My]
  Mux1/1 -> Product1/3
  [Cm_T] -> Product3/1
  [Cn_T] -> Product4/1
  Constant4/1 -> Product4/2
  Constant2/1 -> Product2/2
  Input10/1 -> [d_h]
  [d_h] -> Cm/8(Input3)
  [d_h] -> Cn/9(Input4)
  [d_h] -> "Cl "/8(Input4)
  Input11/1 -> [d_a]
  [d_a] -> Cn/10(Input9)
  [d_a] -> "Cl "/9(Input8)

== system f16_6dof3/ 6-DOF Dynamics Model of the F-16/Gravitional Force ==
  Input : Inport
  Constant : Constant  Value=Mass
  Demux : Demux  Outputs=3
  Product : Product
  Output : Outport
  Output1 : Outport  Port=2
  Output2 : Outport  Port=3
  wires:
  Input/1 -> [G_body]
  Constant/1 -> Product/2
  Product/1 -> Demux/1
  Demux/1 -> [F_Gravity_x]
  Demux/2 -> [F_Gravity_y]
  Demux/3 -> [F_Gravity_z]
  [F_Gravity_x] -> Output/1
  [F_Gravity_y] -> Output1/1
  [F_Gravity_z] -> Output2/1
  [G_body] -> Product/1

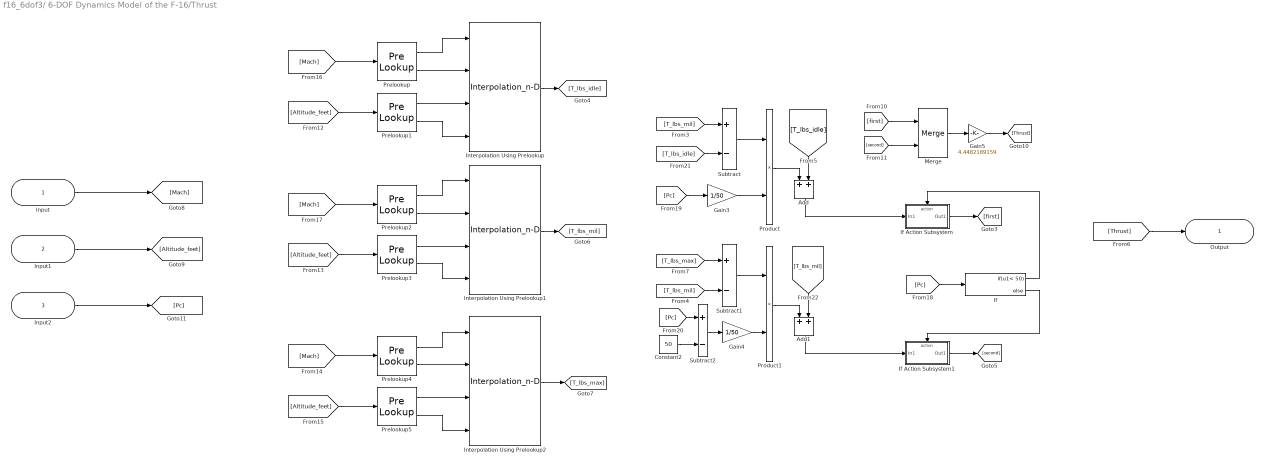
== system f16_6dof3/ 6-DOF Dynamics Model of the F-16/Thrust ==
  Input : Inport
  Input1 : Inport  Port=2
  Input2 : Inport  Port=3
  Add : Sum
  Add1 : Sum
  Constant2 : Constant  Value=50
  Gain3 : Gain  Gain=1/50
  Gain4 : Gain  Gain=1/50
  Gain5 : Gain  Gain=4.4482189159
  If : If  IfExpression=u1< 50
  If Action Subsystem : Subsystem  TreatAsAtomicUnit=on
  If Action Subsystem1 : Subsystem  TreatAsAtomicUnit=on
  Interpolation Using Prelookup : Interpolation_n-D  Table=f16_database.Engine.f16_EngineData.data.Thrust_lbs.idle  InternalRulePriority=Speed
  Interpolation Using Prelookup1 : Interpolation_n-D  Table=f16_database.Engine.f16_EngineData.data.Thrust_lbs.mil  InternalRulePriority=Speed
  Interpolation Using Prelookup2 : Interpolation_n-D  Table=f16_database.Engine.f16_EngineData.data.Thrust_lbs.max  InternalRulePriority=Speed
  Merge : Merge
  Prelookup : PreLookup  BreakpointsData=f16_database.Engine.f16_EngineData.BP.idle.mach  ExtrapMethod=Linear
  Prelookup1 : PreLookup  BreakpointsData=f16_database.Engine.f16_EngineData.BP.idle.alt_ft  ExtrapMethod=Linear
  Prelookup2 : PreLookup  BreakpointsData=f16_database.Engine.f16_EngineData.BP.mil.mach  ExtrapMethod=Linear
  Prelookup3 : PreLookup  BreakpointsData=f16_database.Engine.f16_EngineData.BP.mil.alt_ft  ExtrapMethod=Linear
  Prelookup4 : PreLookup  BreakpointsData=f16_database.Engine.f16_EngineData.BP.max.mach  ExtrapMethod=Linear
  Prelookup5 : PreLookup  BreakpointsData=f16_database.Engine.f16_EngineData.BP.max.alt_ft  ExtrapMethod=Linear
  Product : Product
  Product1 : Product
  Subtract : Sum  Inputs=+-
  Subtract1 : Sum  Inputs=+-
  Subtract2 : Sum  Inputs=+-
  Output : Outport
  wires:
  Prelookup5/1 -> Interpolation Using Prelookup2/3
  Prelookup4/2 -> Interpolation Using Prelookup2/2
  Prelookup3/2 -> Interpolation Using Prelookup1/4
  Interpolation Using Prelookup2/1 -> [T_lbs_max]
  [Mach] -> Prelookup4/1
  [Altitude_feet] -> Prelookup5/1
  [Mach] -> Prelookup/1
  Prelookup5/2 -> Interpolation Using Prelookup2/4
  Prelookup4/1 -> Interpolation Using Prelookup2/1
  Interpolation Using Prelookup1/1 -> [T_lbs_mil]
  Prelookup3/1 -> Interpolation Using Prelookup1/3
  Prelookup2/1 -> Interpolation Using Prelookup1/1
  Prelookup2/2 -> Interpolation Using Prelookup1/2
  [Altitude_feet] -> Prelookup3/1
  [Mach] -> Prelookup2/1
  Prelookup1/2 -> Interpolation Using Prelookup/4
  [Altitude_feet] -> Prelookup1/1
  Prelookup/2 -> Interpolation Using Prelookup/2
  Prelookup/1 -> Interpolation Using Prelookup/1
  Interpolation Using Prelookup/1 -> [T_lbs_idle]
  Prelookup1/1 -> Interpolation Using Prelookup/3
  [T_lbs_mil] -> Subtract/1
  [T_lbs_idle] -> Subtract/2
  [Pc] -> Gain3/1
  Subtract/1 -> Product/1
  Gain3/1 -> Product/2
  Product/1 -> Add/1
  [T_lbs_idle] -> Add/2
  [T_lbs_mil] -> Add1/2
  Product1/1 -> Add1/1
  Gain4/1 -> Product1/2
  Subtract1/1 -> Product1/1
  [T_lbs_mil] -> Subtract1/2
  [T_lbs_max] -> Subtract1/1
  [Pc] -> Subtract2/1
  Constant2/1 -> Subtract2/2
  Subtract2/1 -> Gain4/1
  Add/1 -> If Action Subsystem/1(In1)
  Add1/1 -> If Action Subsystem1/1(In1)
  If Action Subsystem1/1(Out1) -> [second]
  If Action Subsystem/1(Out1) -> [first]
  [Pc] -> If/1
  If/1 -> If Action Subsystem/Action
  If/2 -> If Action Subsystem1/Action
  [Thrust] -> Output/1
  Input/1 -> [Mach]
  Input1/1 -> [Altitude_feet]
  [second] -> Merge/2
  [first] -> Merge/1
  Merge/1 -> Gain5/1
  Input2/1 -> [Pc]
  Gain5/1 -> [Thrust]

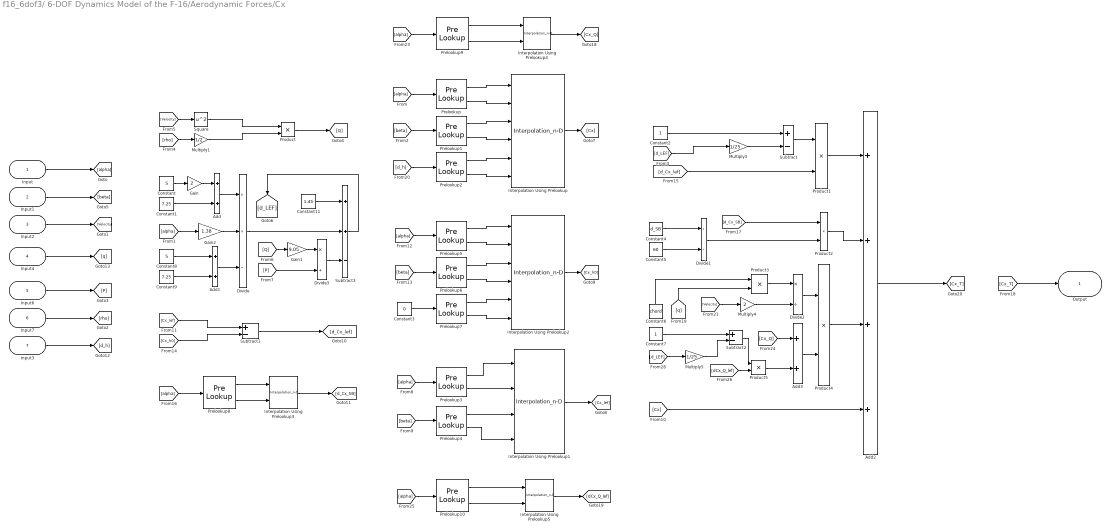
== system f16_6dof3/ 6-DOF Dynamics Model of the F-16/Aerodynamic Forces/Cx ==
  Input : Inport
  Input1 : Inport  Port=2
  Input2 : Inport  Port=3
  Input4 : Inport  Port=4
  Input6 : Inport  Port=5
  Input7 : Inport  Port=6
  Input3 : Inport  Port=7
  Add : Sum
  Add1 : Sum
  Add2 : Sum  Inputs=++++
  Add3 : Sum
  Constant : Constant  Value=S
  Constant1 : Constant  Value=7.25
  Constant11 : Constant  Value=1.45
  Constant2 : Constant
  Constant3 : Constant  Value=0
  Constant4 : Constant  Value=d_SB
  Constant5 : Constant  Value=60
  Constant6 : Constant  Value=chord
  Constant7 : Constant
  Constant8 : Constant  Value=S
  Constant9 : Constant  Value=7.25
  Divide : Product  Inputs=**/
  Divide1 : Product  Inputs=*/
  Divide2 : Product  Inputs=*/
  Divide3 : Product  Inputs=*/
  Gain : Gain  Gain=2
  Gain1 : Gain  Gain=9.05
  Gain2 : Gain  Gain=1.38
  Interpolation Using Prelookup : Interpolation_n-D  NumberOfTableDimensions=3  Table=f16_database.f16_AerodynamicData.data.CX.CX  InternalRulePriority=Speed
      settings: InputPortMap=u0,u1,u2,u3,u4,u5
  Interpolation Using Prelookup1 : Interpolation_n-D  Table=f16_database.f16_AerodynamicData.data.CX.CXlef  InternalRulePriority=Speed
  Interpolation Using Prelookup2 : Interpolation_n-D  NumberOfTableDimensions=3  Table=f16_database.f16_AerodynamicData.data.CX.CX  InternalRulePriority=Speed
      settings: InputPortMap=u0,u1,u2,u3,u4,u5
  Interpolation Using Prelookup3 : Interpolation_n-D  NumberOfTableDimensions=1  Table=f16_database.f16_AerodynamicData.data.CX.deltaCXSB  InternalRulePriority=Speed
      settings: InputPortMap=u0,u1
  Interpolation Using Prelookup4 : Interpolation_n-D  NumberOfTableDimensions=1  Table=f16_database.f16_AerodynamicData.data.CX.CXq  InternalRulePriority=Speed
      settings: InputPortMap=u0,u1
  Interpolation Using Prelookup5 : Interpolation_n-D  NumberOfTableDimensions=1  Table=f16_database.f16_AerodynamicData.data.CX.deltaCXqlef  InternalRulePriority=Speed
      settings: InputPortMap=u0,u1
  Multiply1 : Gain  Gain=1/2
  Multiply3 : Gain  Gain=1/25
  Multiply4 : Gain  Gain=2
  Multiply5 : Gain  Gain=1/25
  Prelookup : PreLookup  BreakpointsData=f16_database.f16_AerodynamicData.BP.CX.CX.alpha  ExtrapMethod=Linear
  Prelookup1 : PreLookup  BreakpointsData=f16_database.f16_AerodynamicData.BP.CX.CX.beta  ExtrapMethod=Linear
  Prelookup10 : PreLookup  BreakpointsData=f16_database.f16_AerodynamicData.BP.CX.deltaCXqlef.alpha  ExtrapMethod=Linear
  Prelookup2 : PreLookup  BreakpointsData=f16_database.f16_AerodynamicData.BP.CX.CX.dHT  ExtrapMethod=Linear
  Prelookup3 : PreLookup  BreakpointsData=f16_database.f16_AerodynamicData.BP.CX.CXlef.alpha  ExtrapMethod=Linear
  Prelookup4 : PreLookup  BreakpointsData=f16_database.f16_AerodynamicData.BP.CX.CXlef.beta  ExtrapMethod=Linear
  Prelookup5 : PreLookup  BreakpointsData=f16_database.f16_AerodynamicData.BP.CX.CX.alpha  ExtrapMethod=Linear
  Prelookup6 : PreLookup  BreakpointsData=f16_database.f16_AerodynamicData.BP.CX.CX.beta  ExtrapMethod=Linear
  Prelookup7 : PreLookup  BreakpointsData=f16_database.f16_AerodynamicData.BP.CX.CX.dHT  ExtrapMethod=Linear
  Prelookup8 : PreLookup  BreakpointsData=f16_database.f16_AerodynamicData.BP.CX.deltaCXSB.alpha  ExtrapMethod=Linear
  Prelookup9 : PreLookup  BreakpointsData=f16_database.f16_AerodynamicData.BP.CX.CXq.alpha  ExtrapMethod=Linear
  Product{,1..5} (6 alike) : Product
  Square : Math  Operator=square  SaturateOnIntegerOverflow=on
  Subtract : Sum  Inputs=+-
  Subtract1 : Sum  Inputs=+-
  Subtract2 : Sum  Inputs=+-
  Subtract3 : Sum  Inputs=++-
  Output : Outport
  wires:
  [Cx_Q] -> Add3/1
  Constant4/1 -> Divide1/1
  Prelookup3/2 -> Interpolation Using Prelookup1/2
  Prelookup10/1 -> Interpolation Using Prelookup5/1
  Prelookup4/1 -> Interpolation Using Prelookup1/3
  Prelookup8/2 -> Interpolation Using Prelookup3/2
  Prelookup/1 -> Interpolation Using Prelookup/1
  [Velocity] -> Square/1
  Prelookup2/2 -> Interpolation Using Prelookup/6
  [alpha] -> Prelookup8/1
  Prelookup8/1 -> Interpolation Using Prelookup3/1
  [alpha] -> Prelookup/1
  Prelookup9/1 -> Interpolation Using Prelookup4/1
  Prelookup3/1 -> Interpolation Using Prelookup1/1
  Multiply4/1 -> Divide2/2
  [beta] -> Prelookup4/1
  [alpha] -> Prelookup3/1
  [Cx_h0] -> Subtract1/2
  [d_Cx_SB] -> Product2/1
  Add3/1 -> Product4/2
  Prelookup5/1 -> Interpolation Using Prelookup2/1
  Prelookup7/1 -> Interpolation Using Prelookup2/5
  Divide1/1 -> Product2/2
  Prelookup9/2 -> Interpolation Using Prelookup4/2
  Prelookup4/2 -> Interpolation Using Prelookup1/4
  Prelookup2/1 -> Interpolation Using Prelookup/5
  Prelookup6/2 -> Interpolation Using Prelookup2/4
  Interpolation Using Prelookup1/1 -> [Cx_lef]
  [d_h] -> Prelookup2/1
  [alpha] -> Prelookup5/1
  Subtract1/1 -> [d_Cx_lef]
  Prelookup1/1 -> Interpolation Using Prelookup/3
  Multiply1/1 -> Product/2
  Product1/1 -> Add2/1
  Prelookup5/2 -> Interpolation Using Prelookup2/2
  [beta] -> Prelookup1/1
  Add2/1 -> [Cx_T]
  Constant5/1 -> Divide1/2
  Product/1 -> [Q]
  Constant6/1 -> Product3/1
  [d_LEF] -> Multiply3/1
  Interpolation Using Prelookup2/1 -> [Cx_h0]
  Interpolation Using Prelookup5/1 -> [dCx_Q_lef]
  Interpolation Using Prelookup3/1 -> [d_Cx_SB]
  Prelookup10/2 -> Interpolation Using Prelookup5/2
  [alpha] -> Prelookup10/1
  [rho] -> Multiply1/1
  [d_Cx_lef] -> Product1/2
  Constant3/1 -> Prelookup7/1
  Prelookup1/2 -> Interpolation Using Prelookup/4
  [Velocity] -> Multiply4/1
  Interpolation Using Prelookup/1 -> [Cx]
  Prelookup7/2 -> Interpolation Using Prelookup2/6
  Subtract/1 -> Product1/1
  Prelookup6/1 -> Interpolation Using Prelookup2/3
  Prelookup/2 -> Interpolation Using Prelookup/2
  Constant2/1 -> Subtract/1
  Product3/1 -> Divide2/1
  Multiply3/1 -> Subtract/2
  Divide2/1 -> Product4/1
  [d_LEF] -> Multiply5/1
  Multiply5/1 -> Subtract2/2
  [alpha] -> Prelookup9/1
  Interpolation Using Prelookup4/1 -> [Cx_Q]
  Constant7/1 -> Subtract2/1
  [dCx_Q_lef] -> Product5/2
  Subtract2/1 -> Product5/1
  [q] -> Product3/2
  [beta] -> Prelookup6/1
  Product5/1 -> Add3/2
  Square/1 -> Product/1
  [Cx_lef] -> Subtract1/1
  Input/1 -> [alpha]
  Input6/1 -> [P]
  Input7/1 -> [rho]
  Input4/1 -> [q]
  Input2/1 -> [Velocity]
  Input1/1 -> [beta]
  [Cx_T] -> Output/1
  Product4/1 -> Add2/3
  [Cx] -> Add2/4
  Product2/1 -> Add2/2
  Input3/1 -> [d_h]
  Constant/1 -> Gain/1
  Gain/1 -> Add/1
  Constant1/1 -> Add/2
  Constant8/1 -> Add1/1
  Constant9/1 -> Add1/2
  Add/1 -> Divide/1
  Add1/1 -> Divide/3
  [alpha] -> Gain2/1
  Gain2/1 -> Divide/2
  Divide/1 -> Subtract3/2
  [P] -> Divide3/2
  [Q] -> Gain1/1
  Gain1/1 -> Divide3/1
  Divide3/1 -> Subtract3/3
  Constant11/1 -> Subtract3/1
  Subtract3/1 -> [d_LEF]

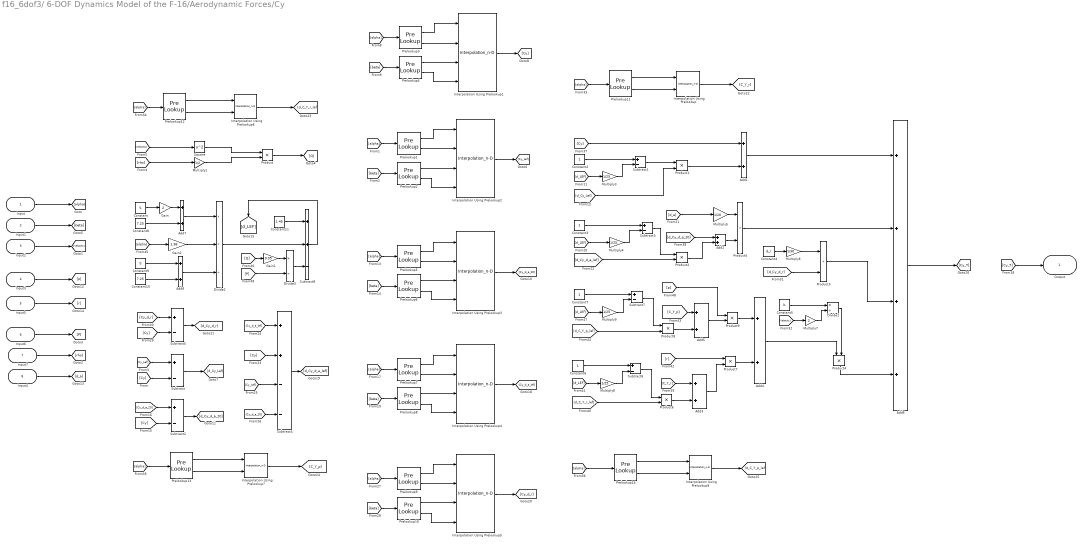
== system f16_6dof3/ 6-DOF Dynamics Model of the F-16/Aerodynamic Forces/Cy ==
  Input : Inport
  Input1 : Inport  Port=2
  Input2 : Inport  Port=3
  Input3 : Inport  Port=4
  Input5 : Inport  Port=5
  Input6 : Inport  Port=6
  Input7 : Inport  Port=7
  Input4 : Inport  Port=8
  Add{1..5,7..8} (7 alike) : Sum
  Add6 : Sum  Inputs=++++
  Constant : Constant  Value=S
  Constant10 : Constant  Value=7.25
  Constant11 : Constant  Value=1.45
  Constant{2..3,6..7} (4 alike) : Constant
  Constant4 : Constant  Value=d_r
  Constant5 : Constant  Value=b
  Constant8 : Constant  Value=7.25
  Constant9 : Constant  Value=S
  Divide1 : Product  Inputs=*/
  Divide2 : Product  Inputs=**/
  Divide3 : Product  Inputs=*/
  Gain : Gain  Gain=2
  Gain1 : Gain  Gain=9.05
  Gain2 : Gain  Gain=1.38
  Interpolation Using Prelookup : Interpolation_n-D  NumberOfTableDimensions=1  Table=f16_database.f16_AerodynamicData.data.CY.CYr  InternalRulePriority=Speed
      settings: InputPortMap=u0,u1
  Interpolation Using Prelookup1 : Interpolation_n-D  Table=f16_database.f16_AerodynamicData.data.CY.CY  InternalRulePriority=Speed
  Interpolation Using Prelookup2 : Interpolation_n-D  Table=f16_database.f16_AerodynamicData.data.CY.CYlef  InternalRulePriority=Speed
  Interpolation Using Prelookup3 : Interpolation_n-D  Table=f16_database.f16_AerodynamicData.data.CY.CYda20  InternalRulePriority=Speed
  Interpolation Using Prelookup4 : Interpolation_n-D  Table=f16_database.f16_AerodynamicData.data.CY.CYda20lef  InternalRulePriority=Speed
  Interpolation Using Prelookup5 : Interpolation_n-D  Table=f16_database.f16_AerodynamicData.data.CY.CYdr30  InternalRulePriority=Speed
  Interpolation Using Prelookup6 : Interpolation_n-D  NumberOfTableDimensions=1  Table=f16_database.f16_AerodynamicData.data.CY.deltaCYrlef  InternalRulePriority=Speed
      settings: InputPortMap=u0,u1
  Interpolation Using Prelookup7 : Interpolation_n-D  NumberOfTableDimensions=1  Table=f16_database.f16_AerodynamicData.data.CY.CYp  InternalRulePriority=Speed
      settings: InputPortMap=u0,u1
  Interpolation Using Prelookup8 : Interpolation_n-D  NumberOfTableDimensions=1  Table=f16_database.f16_AerodynamicData.data.CY.deltaCYplef  InternalRulePriority=Speed
      settings: InputPortMap=u0,u1
  Multiply1 : Gain  Gain=1/2
  Multiply{3..4,8..9} (4 alike) : Gain  Gain=1/25
  Multiply5 : Gain  Gain=1/20
  Multiply6 : Gain  Gain=1/30
  Multiply7 : Gain  Gain=2
  Prelookup1 : PreLookup  BreakpointsData=f16_database.f16_AerodynamicData.BP.CY.CYlef.alpha  ExtrapMethod=Linear
  Prelookup10 : PreLookup  BreakpointsData=f16_database.f16_AerodynamicData.BP.CY.CYdr30.beta  ExtrapMethod=Linear
  Prelookup11 : PreLookup  BreakpointsData=f16_database.f16_AerodynamicData.BP.CY.CYr.alpha  ExtrapMethod=Linear
  Prelookup12 : PreLookup  BreakpointsData=f16_database.f16_AerodynamicData.BP.CY.deltaCYrlef.alpha  ExtrapMethod=Linear
  Prelookup13 : PreLookup  BreakpointsData=f16_database.f16_AerodynamicData.BP.CY.CYp.alpha  ExtrapMethod=Linear
  Prelookup14 : PreLookup  BreakpointsData=f16_database.f16_AerodynamicData.BP.CY.deltaCYplef.alpha  ExtrapMethod=Linear
  Prelookup2 : PreLookup  BreakpointsData=f16_database.f16_AerodynamicData.BP.CY.CYlef.beta  ExtrapMethod=Linear
  Prelookup3 : PreLookup  BreakpointsData=f16_database.f16_AerodynamicData.BP.CY.CY.alpha  ExtrapMethod=Linear
  Prelookup4 : PreLookup  BreakpointsData=f16_database.f16_AerodynamicData.BP.CY.CY.beta  ExtrapMethod=Linear
  Prelookup5 : PreLookup  BreakpointsData=f16_database.f16_AerodynamicData.BP.CY.CYda20.alpha  ExtrapMethod=Linear
  Prelookup6 : PreLookup  BreakpointsData=f16_database.f16_AerodynamicData.BP.CY.CYda20.beta  ExtrapMethod=Linear
  Prelookup7 : PreLookup  BreakpointsData=f16_database.f16_AerodynamicData.BP.CY.CYda20lef.alpha  ExtrapMethod=Linear
  Prelookup8 : PreLookup  BreakpointsData=f16_database.f16_AerodynamicData.BP.CY.CYda20lef.beta  ExtrapMethod=Linear
  Prelookup9 : PreLookup  BreakpointsData=f16_database.f16_AerodynamicData.BP.CY.CYdr30.alpha  ExtrapMethod=Linear
  Product{,1..9} (10 alike) : Product
  Square : Math  Operator=square  SaturateOnIntegerOverflow=on
  Subtract{,1..3,5..7} (7 alike) : Sum  Inputs=+-
  Subtract4 : Sum  Inputs=++--
  Subtract8 : Sum  Inputs=++-
  Output : Outport
  wires:
  Prelookup3/2 -> Interpolation Using Prelookup1/2
  Prelookup4/1 -> Interpolation Using Prelookup1/3
  [Velocity] -> Square/1
  Prelookup3/1 -> Interpolation Using Prelookup1/1
  [beta] -> Prelookup4/1
  [alpha] -> Prelookup3/1
  Prelookup4/2 -> Interpolation Using Prelookup1/4
  Interpolation Using Prelookup1/1 -> [Cy]
  Multiply1/1 -> Product/2
  Product/1 -> [Q]
  [rho] -> Multiply1/1
  Square/1 -> Product/1
  Input/1 -> [alpha]
  Input3/1 -> [p]
  Input5/1 -> [r]
  Input6/1 -> [P]
  Input7/1 -> [rho]
  Input2/1 -> [Velocity]
  Input1/1 -> [beta]
  [Cy_T] -> Output/1
  Prelookup1/2 -> Interpolation Using Prelookup2/2
  [alpha] -> Prelookup1/1
  Prelookup2/2 -> Interpolation Using Prelookup2/4
  Prelookup1/1 -> Interpolation Using Prelookup2/1
  [beta] -> Prelookup2/1
  Prelookup2/1 -> Interpolation Using Prelookup2/3
  Interpolation Using Prelookup2/1 -> [Cy_Lef]
  [Cy_Lef] -> Subtract/1
  [Cy] -> Subtract/2
  Subtract/1 -> [d_Cy_Lef]
  [d_LEF] -> Multiply3/1
  [d_Cy_Lef] -> Product1/2
  Constant2/1 -> Subtract1/1
  Multiply3/1 -> Subtract1/2
  Subtract1/1 -> Product1/1
  Interpolation Using Prelookup3/1 -> [Cy_d_a_20]
  Prelookup6/1 -> Interpolation Using Prelookup3/3
  [beta] -> Prelookup6/1
  Prelookup5/1 -> Interpolation Using Prelookup3/1
  Prelookup6/2 -> Interpolation Using Prelookup3/4
  [alpha] -> Prelookup5/1
  Prelookup5/2 -> Interpolation Using Prelookup3/2
  [Cy_d_a_20] -> Subtract2/1
  [Cy] -> Subtract2/2
  Subtract2/1 -> [d_Cy_d_a_20]
  Prelookup7/2 -> Interpolation Using Prelookup4/2
  [alpha] -> Prelookup7/1
  Prelookup8/2 -> Interpolation Using Prelookup4/4
  Prelookup7/1 -> Interpolation Using Prelookup4/1
  [beta] -> Prelookup8/1
  Prelookup8/1 -> Interpolation Using Prelookup4/3
  Interpolation Using Prelookup4/1 -> [Cy_d_a_lef]
  Subtract3/1 -> Product2/1
  [d_LEF] -> Multiply4/1
  Multiply4/1 -> Subtract3/2
  Product2/1 -> Add2/2
  [d_Cy_d_a_lef] -> Product2/2
  Constant3/1 -> Subtract3/1
  Subtract4/1 -> [d_Cy_d_a_lef]
  [d_a] -> Multiply5/1
  [Cy_d_a_lef] -> Subtract4/1
  [Cy_Lef] -> Subtract4/3
  [Cy_d_a_20] -> Subtract4/4
  [Cy] -> Subtract4/2
  Prelookup9/2 -> Interpolation Using Prelookup5/2
  Interpolation Using Prelookup5/1 -> [Cy_d_r]
  Prelookup10/1 -> Interpolation Using Prelookup5/3
  Prelookup10/2 -> Interpolation Using Prelookup5/4
  [beta] -> Prelookup10/1
  [alpha] -> Prelookup9/1
  Prelookup9/1 -> Interpolation Using Prelookup5/1
  Subtract5/1 -> [d_Cy_d_r]
  [Cy] -> Subtract5/2
  [Cy_d_r] -> Subtract5/1
  Constant4/1 -> Multiply6/1
  Multiply6/1 -> Product3/1
  [d_Cy_d_r] -> Product3/2
  Constant5/1 -> Divide1/1
  [Velocity] -> Multiply7/1
  Multiply7/1 -> Divide1/2
  [alpha] -> Prelookup11/1
  Prelookup11/1 -> Interpolation Using Prelookup/1
  Prelookup11/2 -> Interpolation Using Prelookup/2
  Interpolation Using Prelookup/1 -> [C_Y_r]
  Interpolation Using Prelookup6/1 -> [d_C_Y_r_lef]
  Prelookup12/2 -> Interpolation Using Prelookup6/2
  Prelookup12/1 -> Interpolation Using Prelookup6/1
  [alpha] -> Prelookup12/1
  [alpha] -> Prelookup13/1
  Prelookup13/1 -> Interpolation Using Prelookup7/1
  Prelookup13/2 -> Interpolation Using Prelookup7/2
  Interpolation Using Prelookup7/1 -> [C_Y_p]
  Interpolation Using Prelookup8/1 -> [d_C_Y_p_lef]
  Prelookup14/2 -> Interpolation Using Prelookup8/2
  Prelookup14/1 -> Interpolation Using Prelookup8/1
  [alpha] -> Prelookup14/1
  [Cy] -> Add1/1
  Product1/1 -> Add1/2
  [d_Cy_d_a_20] -> Add2/1
  Add2/1 -> Product5/2
  Multiply5/1 -> Product5/1
  Constant6/1 -> Subtract6/1
  [d_LEF] -> Multiply8/1
  Subtract6/1 -> Product6/1
  Multiply8/1 -> Subtract6/2
  [d_C_Y_r_lef] -> Product6/2
  [C_Y_r] -> Add3/1
  Product6/1 -> Add3/2
  Add3/1 -> Product7/2
  [r] -> Product7/1
  Product7/1 -> Add4/2
  [p] -> Product9/1
  Add5/1 -> Product9/2
  Product8/1 -> Add5/2
  [C_Y_p] -> Add5/1
  [d_C_Y_p_lef] -> Product8/2
  Multiply9/1 -> Subtract7/2
  Subtract7/1 -> Product8/1
  [d_LEF] -> Multiply9/1
  Constant7/1 -> Subtract7/1
  Product9/1 -> Add4/1
  Divide1/1 -> Product4/2
  Add4/1 -> Product4/1
  Add1/1 -> Add6/1
  Product5/1 -> Add6/2
  Product4/1 -> Add6/4
  Product3/1 -> Add6/3
  Add6/1 -> [Cy_T]
  Input4/1 -> [d_a]
  [P] -> Divide3/2
  Gain/1 -> Add7/1
  Divide3/1 -> Subtract8/3
  Divide2/1 -> Subtract8/2
  Subtract8/1 -> [d_LEF]
  Constant10/1 -> Add8/2
  Gain1/1 -> Divide3/1
  [alpha] -> Gain2/1
  Constant9/1 -> Add8/1
  [Q] -> Gain1/1
  Constant8/1 -> Add7/2
  Gain2/1 -> Divide2/2
  Constant/1 -> Gain/1
  Constant11/1 -> Subtract8/1
  Add8/1 -> Divide2/3
  Add7/1 -> Divide2/1
